simulink model "MagneticFieldInPolarCoords"  (R2020b)
settings: Solver=VariableStepAuto  StartTime=0.0  StopTime=10.0  RelTol=1e-3
settings Model: Creator=matteo  LastModifiedBy=matteo

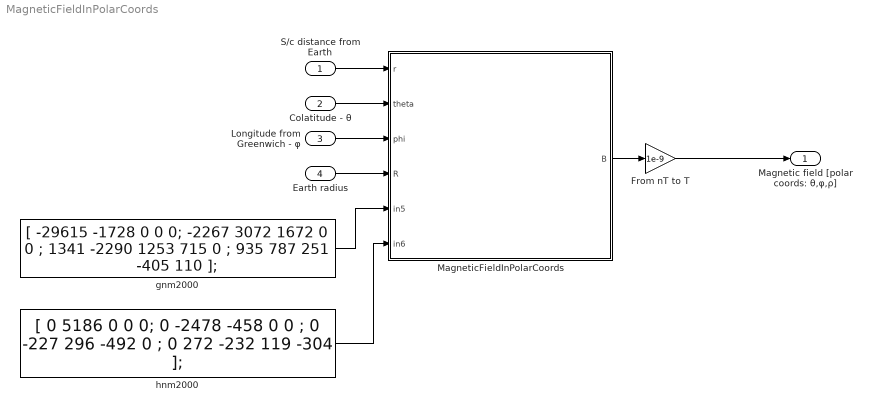
== system MagneticFieldInPolarCoords ==
  S/c distance from Earth : Inport
  Colatitude - θ : Inport  Port=2
  Longitude from Greenwich - φ : Inport  Port=3
  Earth radius : Inport  Port=4
  From nT to T : Gain  Gain=1e-9
  MagneticFieldInPolarCoords : MATLAB Function  TreatAsAtomicUnit=on
  gnm2000 : Constant  Value=|
      | [ -29615  -1728      0      0      0;
      | -2267   3072   1672      0      0 ;
      | 1341  -2290   1253    715      0 ;  935    787    251   -405    110 ];
  hnm2000 : Constant  Value="[      0   5186      0      0      0; 0  -2478   -458      0      0 ; 0   -227    296   -492      0 ; 0    272   -232    119   -304 ];"
  Magnetic field [polar coords: θ,φ,ρ] : Outport
  wires:
  Colatitude - θ/1 -> MagneticFieldInPolarCoords/2(theta)
  gnm2000/1 -> MagneticFieldInPolarCoords/5(in5)
  Earth radius/1 -> MagneticFieldInPolarCoords/4(R)
  hnm2000/1 -> MagneticFieldInPolarCoords/6(in6)
  Longitude from Greenwich - φ/1 -> MagneticFieldInPolarCoords/3(phi)
  MagneticFieldInPolarCoords/1(B) -> From nT to T/1
  From nT to T/1 -> Magnetic field [polar coords: θ,φ,ρ]/1
  S/c distance from Earth/1 -> MagneticFieldInPolarCoords/1(r)

== matlab function MagneticFieldInPolarCoords/MagneticFieldInPolarCoords ==
  data: r input; B output; theta input; phi input; R input; in5 input; in6 input
function B = MagneticFieldInPolarCoords(r,theta,phi,R,in5,in6)
%#codegen

%    This function was generated by the Symbolic Math Toolbox version 8.6.
%    21-Nov-2020 10:08:44

g_1_1 = in5(1);
g_1_2 = in5(5);
g_2_1 = in5(2);
g_2_2 = in5(6);
g_2_3 = in5(10);
g_3_1 = in5(3);
g_3_2 = in5(7);
g_3_3 = in5(11);
g_3_4 = in5(15);
g_4_1 = in5(4);
g_4_2 = in5(8);
g_4_3 = in5(12);
g_4_4 = in5(16);
g_4_5 = in5(20);
h_1_2 = in6(5);
h_2_2 = in6(6);
h_2_3 = in6(10);
h_3_2 = in6(7);
h_3_3 = in6(11);
h_3_4 = in6(15);
h_4_2 = in6(8);
h_4_3 = in6(12);
h_4_4 = in6(16);
h_4_5 = in6(20);
t2 = cos(phi);
t3 = cos(theta);
t4 = sin(phi);
t5 = sin(theta);
t6 = R.^3;
t7 = R.^4;
t8 = R.^5;
t10 = phi.*2.0;
t11 = phi.*3.0;
t12 = phi.*4.0;
t24 = 1.0./r;
t30 = sqrt(2.0);
t31 = sqrt(3.0);
t32 = sqrt(5.0);
t35 = sqrt(1.5e+1);
t36 = sqrt(3.5e+1);
t9 = t6.^2;
t13 = cos(t10);
t14 = cos(t11);
t15 = cos(t12);
t16 = t3.^2;
t17 = t3.^3;
t18 = sin(t10);
t19 = sin(t11);
t20 = sin(t12);
t21 = t5.^2;
t22 = t5.^3;
t25 = t24.^3;
t26 = t24.^4;
t27 = t24.^5;
t29 = 1.0./t5;
t33 = t3./5.0;
t34 = t5./5.0;
t37 = g_1_2.*t2.*t5;
t39 = t3.*(4.0./1.5e+1);
t40 = t5.*(4.0./1.5e+1);
t44 = t3.*t5.*(2.0./7.0);
t57 = t3.*t5.*(8.0./3.5e+1);
t68 = g_2_2.*t2.*t3.*t5.*t31;
t23 = t21.^2;
t28 = t25.^2;
t38 = t29.*theta;
t41 = t5.*t16;
t42 = -t17;
t43 = -t21;
t45 = -t40;
t46 = t3.*t21.*2.0;
t48 = t3.*t22.*2.0;
t49 = t5.*t17.*2.0;
t50 = t21./7.0;
t55 = t16-1.0./3.0;
t56 = t16.*t21;
t58 = t16.*(8.0./3.5e+1);
t59 = t21.*(8.0./3.5e+1);
t47 = t41.*2.0;
t51 = -t38;
t52 = -t41;
t54 = -t49;
t60 = t56.*3.0;
t62 = -t59;
t63 = t16.*t43;
t65 = t16+t43;
t66 = t3.*t55;
t67 = t5.*t55;
t78 = t33+t42+t46;
t53 = -t47;
t61 = (t51 ~= 0.0);
t64 = -t60;
t70 = -t66;
t71 = t34+t52;
t75 = t50+t63;
t79 = t3.*t78;
t80 = t44+t48+t54;
t81 = t45+t47+t67;
t69 = t22+t53;
t72 = t23+t64;
t73 = t3.*t71;
t74 = t5.*t71;
t77 = t39+t70;
t83 = g_3_2.*t2.*t30.*t31.*t71.*(5.0./4.0);
t76 = -t74;
t82 = t57+t73;
t84 = -t83;
t85 = g_4_2.*t2.*t30.*t32.*t82.*(7.0./4.0);
t86 = t58+t62+t76+t79;
B = [R.*t24.*(-g_1_1.*t5+g_1_2.*t2.*t3+h_1_2.*t3.*t4).*-3.0+R.*t24.*(g_3_1.*t81.*(5.0./2.0)+(g_3_3.*t13.*t35.*t69)./2.0+(h_3_3.*t18.*t35.*t69)./2.0+g_3_2.*t2.*t30.*t31.*t78.*(5.0./4.0)+h_3_2.*t4.*t30.*t31.*t78.*(5.0./4.0)-g_3_4.*t3.*t14.*t21.*t30.*t32.*(3.0./4.0)-h_3_4.*t3.*t19.*t21.*t30.*t32.*(3.0./4.0)).*5.0+R.*t24.*(g_4_1.*(t3.*t5.*(1.8e+1./3.5e+1)+t5.*t77-t3.*t81).*(-3.5e+1./8.0)+g_4_3.*t13.*t32.*t80.*(7.0./4.0)+h_4_3.*t18.*t32.*t80.*(7.0./4.0)-(g_4_5.*t3.*t15.*t22.*t36)./2.0+g_4_2.*t2.*t30.*t32.*t86.*(7.0./4.0)+(g_4_4.*t14.*t30.*t36.*t72)./4.0-(h_4_5.*t3.*t20.*t22.*t36)./2.0+h_4_2.*t4.*t30.*t32.*t86.*(7.0./4.0)+(h_4_4.*t19.*t30.*t36.*t72)./4.0).*6.0-R.*t24.*(g_2_1.*t3.*t5.*-3.0+g_2_2.*t2.*t31.*t65+h_2_2.*t4.*t31.*t65+g_2_3.*t3.*t5.*t13.*t31+h_2_3.*t3.*t5.*t18.*t31).*4.0;t6.*t25.*t61.*(t37-g_1_2.*t4.*t5)+t7.*t26.*t61.*(t68+g_2_3.*t13.*t21.*t31+g_2_3.*t18.*t31.*t43-g_2_2.*t3.*t4.*t5.*t31)+t8.*t27.*t61.*(t84+g_3_3.*t3.*t13.*t21.*t35+g_3_3.*t3.*t18.*t35.*t43+g_3_4.*t14.*t22.*t30.*t32.*(3.0./4.0)-g_3_4.*t19.*t22.*t30.*t32.*(3.0./4.0)+g_3_2.*t4.*t30.*t31.*t71.*(5.0./4.0))-t9.*t28.*t61.*(t85-(g_4_5.*t15.*t23.*t36)./2.0+(g_4_5.*t20.*t23.*t36)./2.0+g_4_3.*t13.*t32.*t75.*(7.0./2.0)-g_4_3.*t18.*t32.*t75.*(7.0./2.0)-g_4_2.*t4.*t30.*t32.*t82.*(7.0./4.0)-g_4_4.*t3.*t14.*t22.*t30.*t36.*(3.0./4.0)+g_4_4.*t3.*t19.*t22.*t30.*t36.*(3.0./4.0));t6.*t25.*(t37+g_1_1.*t3+h_1_2.*t4.*t5).*2.0+t7.*t26.*(t68+g_2_1.*t55.*(3.0./2.0)+(g_2_3.*t13.*t21.*t31)./2.0+(h_2_3.*t18.*t21.*t31)./2.0+h_2_2.*t3.*t4.*t5.*t31).*3.0+t8.*t27.*(t84-g_3_1.*t77.*(5.0./2.0)+(g_3_3.*t3.*t13.*t21.*t35)./2.0+(g_3_4.*t14.*t22.*t30.*t32)./4.0+(h_3_3.*t3.*t18.*t21.*t35)./2.0+(h_3_4.*t19.*t22.*t30.*t32)./4.0-h_3_2.*t4.*t30.*t31.*t71.*(5.0./4.0)).*4.0-t9.*t28.*(t85+g_4_1.*(t16.*(9.0./3.5e+1)+t3.*t77-3.0./3.5e+1).*(3.5e+1./8.0)-(g_4_5.*t15.*t23.*t36)./8.0+g_4_3.*t13.*t32.*t75.*(7.0./4.0)-(h_4_5.*t20.*t23.*t36)./8.0+h_4_3.*t18.*t32.*t75.*(7.0./4.0)+h_4_2.*t4.*t30.*t32.*t82.*(7.0./4.0)-(g_4_4.*t3.*t14.*t22.*t30.*t36)./4.0-(h_4_4.*t3.*t19.*t22.*t30.*t36)./4.0).*5.0];
